simulink model "problem1_1s"  (R2021a)
settings: Solver=FixedStepAuto  StartTime=0.0  StopTime=28.5  FixedStep=0.001  RelTol=1e-3  EnableMultiTasking=on
StopFcn:
  | mypi=raspi();
  | writeDigitalPin(mypi,19,0);
  | writeDigitalPin(mypi,26,0);
  | writeDigitalPin(mypi,20,0);
  | writeDigitalPin(mypi,21,0);
  | clear mypi;
libraries: raspberrypiBasiclib x3
settings Model: Creator=HP  LastModifiedBy=ku347
settings SolverCC: PositivePriorityOrder=on
settings OptimizationCC: EnhancedBackFolding=on  PassReuseOutputArgsAs=Individual arguments  ZeroExternalMemoryAtStartup=off  ZeroInternalMemoryAtStartup=off  MaxStackSize=64  OptimizeBlockOrder=speed  DifferentSizesBufferReuse=on  OptimizationCustomize=off  EfficientTunableParamExpr=on
settings DebuggingCC: ParameterTunabilityLossMsg=error  UnconnectedInputMsg=none  UnconnectedOutputMsg=none  UnconnectedLineMsg=none
settings HardwareCC: ProdBitPerPointer=32  ProdBitPerSizeT=32  ProdBitPerPtrDiffT=32  ProdLargestAtomicInteger=Long  ProdLargestAtomicFloat=Double  ProdWordSize=32  ProdLongLongMode=on  ProdHWDeviceType=ARM Compatible->ARM Cortex  UseEmbeddedCoderFeatures=off
settings RTWCC: SystemTargetFile=ert.tlc  HardwareBoard=Raspberry Pi  TLCOptions="-aInlineSetEventsForThisBaseRateFcn=TLC_FALSE -aSuppressMultiTaskScheduler=TLC_FALSE  -aRateBasedStepFcn=0"  TemplateMakefile=ert_default_tmf  Toolchain=GNU GCC Embedded Linux  BuildConfiguration=Specify  DLArmComputeVersion=20.02.1
settings CodeAppCC: ForceParamTrailComments=on  IgnoreCustomStorageClasses=off  OperatorAnnotations=on  SimulinkDataObjDesc=on  SFDataObjDesc=on  InsertBlockDesc=on
settings ERTTargetCC: SupportNonInlinedSFcns=on  SupportVariableSizeSignals=on  ExtModeTransport=2  ExtModeStaticAlloc=on  ExtModeMexFile=ext_xcp  ExtModeIntrfLevel=Level2 - Open

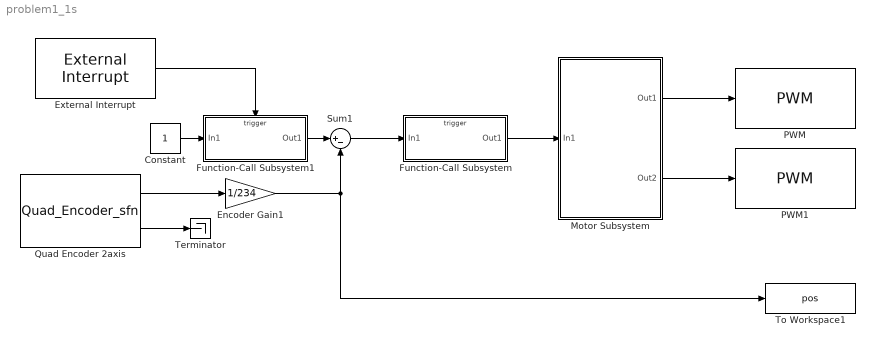
== system problem1_1s ==
  Constant : Constant
  Encoder Gain1 : Gain  Gain=1/234
  External Interrupt : raspberrypiBasiclib/External Interrupt  Board=Pi 4 Model B  Pin=4  PullUp=Pull-down  Mode=Rising  InterruptSimulationInput=off  blockPlatform=Raspberry Pi
      settings: SourceProductBaseCode=RASPPI
  Function-Call Subsystem : Subsystem  TreatAsAtomicUnit=on
  Function-Call Subsystem1 : Subsystem  TreatAsAtomicUnit=on
  Motor Subsystem : Subsystem
  PWM : raspberrypiBasiclib/PWM  board=Pi 4 Model B  Pin_=19  Frequency=1000  blockPlatform=Raspberry Pi
      settings: SourceProductBaseCode=RASPPI
  PWM1 : raspberrypiBasiclib/PWM  board=Pi 4 Model B  Pin_=26  Frequency=1000  blockPlatform=Raspberry Pi
      settings: SourceProductBaseCode=RASPPI
  Quad Encoder 2axis : S-Function  InitFcn=try, set_param(gcb,'FunctionName','Quad_Encoder_sfn'), end  FunctionName=Quad_Encoder_sfn  Parameters=uint8(0),uint8(5),uint8(6),uint8(1),uint8(23),uint8(24)  SFunctionModules=Quad_Encoder_sfn_wrapper  SFunctionDeploymentMode=off  EnableBusSupport=off  mask(S-Function Builder){}
      mask init:
      | val = [[.9  0.75 0.75 1 1 .9 .9 1]',[1 1 0.75 0.75 .9 .9 1 .9]'];try , sys = get_param(gcb,'SfunBuilderFcnName');if isempty(sys), sys = get_param(gcb,'FunctionName'); end,catch, sys = get_param(gcb,'FunctionName'); end
      settings: CopyFcn=set_param(gcbh,'LinkStatus','none')  PreSaveFcn=try, set_param(gcb,'FunctionName','Quad_Encoder_sfn'), end  OpenFcn=sfunctionwizard(gcbh)
      mask Display:
      | plot(val(:,1),val(:,2))
      | disp(sys)
      | port_label('output',1,'enc_pos1')
      | port_label('output',2,'enc_pos2')
  Sum1 : Sum  Inputs=|+-
  Terminator : Terminator
  To Workspace1 : ToWorkspace  VariableName=pos  SampleTime=0.001
  wires:
  Quad Encoder 2axis/1 -> Encoder Gain1/1
  Sum1/1 -> Function-Call Subsystem/1(In1)
  Function-Call Subsystem/1(Out1) -> Motor Subsystem/1(In1)
  Motor Subsystem/1(Out1) -> PWM/1
  Motor Subsystem/2(Out2) -> PWM1/1
  Encoder Gain1/1 -> Sum1/2, To Workspace1/1
  Quad Encoder 2axis/2 -> Terminator/1
  External Interrupt/1 -> Function-Call Subsystem1/Trigger
  Function-Call Subsystem1/1(Out1) -> Sum1/1
  Constant/1 -> Function-Call Subsystem1/1(In1)

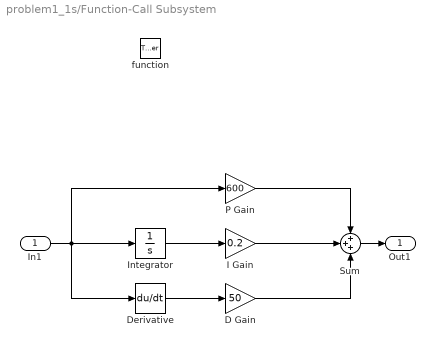
== system problem1_1s/Function-Call Subsystem ==
  In1 : Inport
  function : TriggerPort  TriggerType=function-call  VariantControl=(inherit)
  D Gain : Gain  Gain=50
  Derivative : Derivative
  I Gain : Gain  Gain=0.2
  Integrator : Integrator
  P Gain : Gain  Gain=600
  Sum : Sum  Inputs=+++
  Out1 : Outport
  wires:
  In1/1 -> P Gain/1, Derivative/1, Integrator/1
  Derivative/1 -> D Gain/1
  P Gain/1 -> Sum/1
  Sum/1 -> Out1/1
  Integrator/1 -> I Gain/1
  I Gain/1 -> Sum/2
  D Gain/1 -> Sum/3

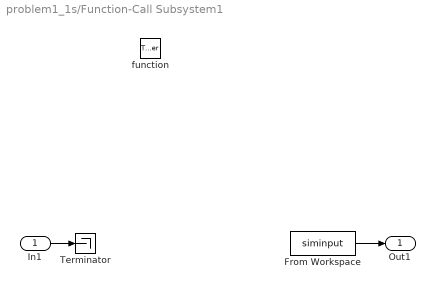
== system problem1_1s/Function-Call Subsystem1 ==
  In1 : Inport
  function : TriggerPort  TriggerType=function-call  VariantControl=(inherit)
  From Workspace : FromWorkspace  VariableName=siminput  SampleTime=0.001
  Terminator : Terminator
  Out1 : Outport
  wires:
  In1/1 -> Terminator/1
  From Workspace/1 -> Out1/1

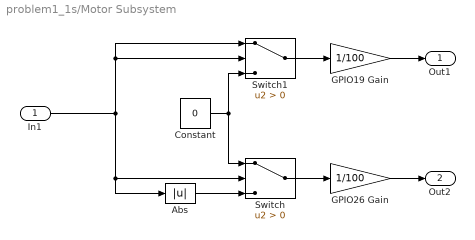
== system problem1_1s/Motor Subsystem ==
  In1 : Inport
  Abs : Abs
  Constant : Constant  Value=0
  GPIO19 Gain : Gain  Gain=1/100
  GPIO26 Gain : Gain  Gain=1/100
  Switch : Switch  Criteria=u2 > Threshold
  Switch1 : Switch  Criteria=u2 > Threshold
  Out1 : Outport
  Out2 : Outport  Port=2
  wires:
  Switch/1 -> GPIO26 Gain/1
  Abs/1 -> Switch/3
  Switch1/1 -> GPIO19 Gain/1
  In1/1 -> Abs/1, Switch/2, Switch1/1, Switch1/2
  Constant/1 -> Switch/1, Switch1/3
  GPIO26 Gain/1 -> Out2/1
  GPIO19 Gain/1 -> Out1/1
